simulink model "B733_SAS"  (R2018a)
settings: Solver=VariableStepAuto  StartTime=0.0  StopTime=S.simtime  RelTol=1e-3
undefined symbols (not defined in the file): S
libraries: peGeneralControl x1
settings Model: Creator=Can Bekar  LastModifiedBy=Can Bekar
settings DataIOCC: ExternalInput=S.usignal  InitialState=xu  LoadExternalInput=on  SignalLogging=off  DSMLogging=off

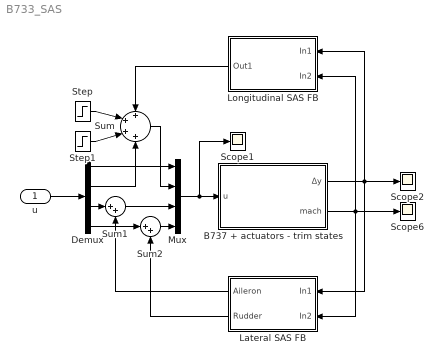
== system B733_SAS ==
  u : Inport
  B737 + actuators - trim states : Subsystem
  Demux : Demux
  Lateral SAS FB : Subsystem
  Longitudinal SAS FB : Subsystem
  Mux : Mux
  Scope1 : Scope
  Scope2 : Scope
  Scope6 : Scope
  Step : Step  Time=2  Before=deg2rad(1)  After=deg2rad(-1)  SampleTime=0
  Step1 : Step  After=deg2rad(1)  SampleTime=0
  Sum : Sum  Inputs=++++
  Sum1 : Sum  Inputs=|++
  Sum2 : Sum  Inputs=|++
  wires:
  Demux/1 -> Mux/1
  Sum/1 -> Mux/2
  Demux/2 -> Sum/4
  Mux/1 -> Scope1/1, B737 + actuators - trim states/1(u)
  u/1 -> Demux/1
  Step1/1 -> Sum/3
  Step/1 -> Sum/2
  Sum1/1 -> Mux/3
  Demux/3 -> Sum1/1
  Sum2/1 -> Mux/4
  Demux/4 -> Sum2/1
  B737 + actuators - trim states/1(Δy) -> Lateral SAS FB/1(In1), Scope2/1, Longitudinal SAS FB/1(In1)
  B737 + actuators - trim states/2(mach) -> Lateral SAS FB/2(In2), Longitudinal SAS FB/2(In2), Scope6/1
  Longitudinal SAS FB/1(Out1) -> Sum/1
  Lateral SAS FB/1(Aileron) -> Sum1/2
  Lateral SAS FB/2(Rudder) -> Sum2/2

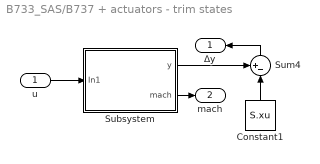
== system B733_SAS/B737 + actuators - trim states ==
  u : Inport
  Constant1 : Constant  Value=S.xu
  Subsystem : Subsystem
  Sum4 : Sum  Inputs=+-|
  Δy : Outport
  mach : Outport  Port=2
  wires:
  Sum4/1 -> Δy/1
  Subsystem/1(y) -> Sum4/1
  u/1 -> Subsystem/1(In1)
  Constant1/1 -> Sum4/2
  Subsystem/2(mach) -> mach/1

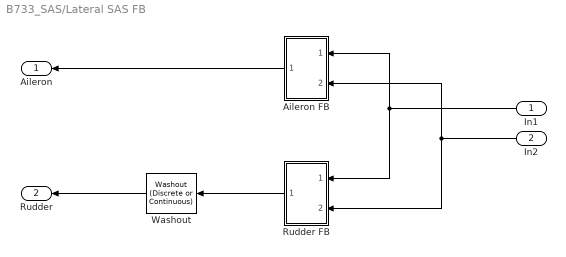
== system B733_SAS/Lateral SAS FB ==
  In1 : Inport
  In2 : Inport  Port=2
  Aileron FB : Subsystem
  Rudder FB : Subsystem
  Washout : peGeneralControl/Washout (Discrete or Continuous)  T=1  Ts=-1
  Aileron : Outport
  Rudder : Outport  Port=2
  wires:
  Washout/1 -> Rudder/1
  In2/1 -> Rudder FB/2(In2), Aileron FB/2(In2)
  In1/1 -> Rudder FB/1(In1), Aileron FB/1(In1)
  Aileron FB/1(Out1) -> Aileron/1
  Rudder FB/1(Out1) -> Washout/1

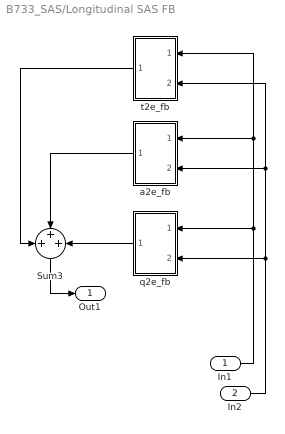
== system B733_SAS/Longitudinal SAS FB ==
  In1 : Inport
  In2 : Inport  Port=2
  Sum3 : Sum  Inputs=+++
  a2e_fb : Subsystem
  q2e_fb : Subsystem
  t2e_fb : Subsystem
  Out1 : Outport
  wires:
  t2e_fb/1(Out1) -> Sum3/1
  Sum3/1 -> Out1/1
  In2/1 -> a2e_fb/2(In2), t2e_fb/2(In2), q2e_fb/2(In2)
  In1/1 -> q2e_fb/1(In1), a2e_fb/1(In1), t2e_fb/1(In1)
  a2e_fb/1(Out1) -> Sum3/2
  q2e_fb/1(Out1) -> Sum3/3

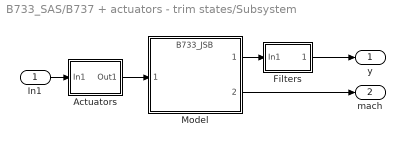
== system B733_SAS/B737 + actuators - trim states/Subsystem ==
  In1 : Inport
  Actuators : Subsystem
  Filters : Subsystem
  Model : ModelReference  ModelNameDialog=B733_JSB  SimulationMode=Normal  ModelReferenceVersion=1.186
  y : Outport
  mach : Outport  Port=2
  wires:
  Model/2 -> mach/1
  Model/1 -> Filters/1(In1)
  Filters/1(Out1) -> y/1
  In1/1 -> Actuators/1(In1)
  Actuators/1(Out1) -> Model/1

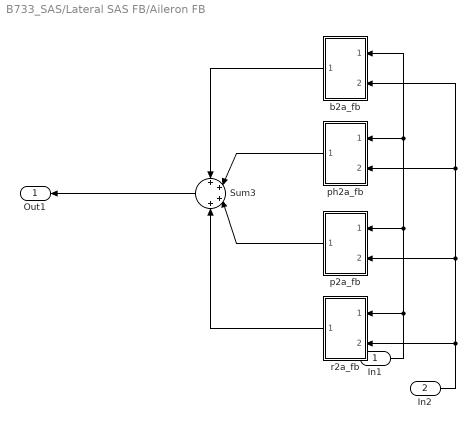
== system B733_SAS/Lateral SAS FB/Aileron FB ==
  In1 : Inport
  In2 : Inport  Port=2
  Sum3 : Sum  Inputs=++++
  b2a_fb : Subsystem
  p2a_fb : Subsystem
  ph2a_fb : Subsystem
  r2a_fb : Subsystem
  Out1 : Outport
  wires:
  p2a_fb/1(Out1) -> Sum3/3
  ph2a_fb/1(Out1) -> Sum3/2
  In2/1 -> b2a_fb/2(In2), ph2a_fb/2(In2), p2a_fb/2(In2), r2a_fb/2(In2)
  b2a_fb/1(Out1) -> Sum3/1
  In1/1 -> b2a_fb/1(In1), ph2a_fb/1(In1), p2a_fb/1(In1), r2a_fb/1(In1)
  r2a_fb/1(Out1) -> Sum3/4
  Sum3/1 -> Out1/1

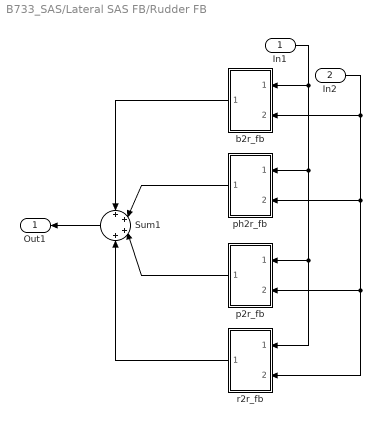
== system B733_SAS/Lateral SAS FB/Rudder FB ==
  In1 : Inport
  In2 : Inport  Port=2
  Sum1 : Sum  Inputs=++++
  b2r_fb : Subsystem
  p2r_fb : Subsystem
  ph2r_fb : Subsystem
  r2r_fb : Subsystem
  Out1 : Outport
  wires:
  r2r_fb/1(Out1) -> Sum1/4
  In2/1 -> ph2r_fb/2(In2), p2r_fb/2(In2), r2r_fb/2(In2), b2r_fb/2(In2)
  b2r_fb/1(Out1) -> Sum1/1
  In1/1 -> ph2r_fb/1(In1), p2r_fb/1(In1), r2r_fb/1(In1), b2r_fb/1(In1)
  p2r_fb/1(Out1) -> Sum1/3
  ph2r_fb/1(Out1) -> Sum1/2
  Sum1/1 -> Out1/1

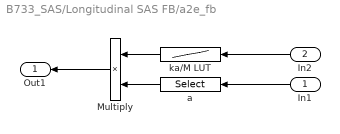
== system B733_SAS/Longitudinal SAS FB/a2e_fb ==
  In1 : Inport
  In2 : Inport  Port=2
  Multiply : Product
  a : Selector  InputPortWidth=12  IndexOptions=Index vector (dialog)  Indices=[2]  OutputSizes=1
  ka/M LUT : Lookup_n-D  NumberOfTableDimensions=1  BreakpointsForDimension1=S.M'  Table=S.kaLUT  InternalRulePriority=Speed  RndMeth=Simplest  InputSameDT=on
  Out1 : Outport
  wires:
  Multiply/1 -> Out1/1
  ka/M LUT/1 -> Multiply/1
  In2/1 -> ka/M LUT/1
  In1/1 -> a/1
  a/1 -> Multiply/2

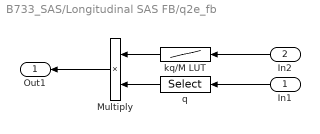
== system B733_SAS/Longitudinal SAS FB/q2e_fb ==
  In1 : Inport
  In2 : Inport  Port=2
  Multiply : Product
  kq/M LUT : Lookup_n-D  NumberOfTableDimensions=1  BreakpointsForDimension1=S.M'  Table=S.kqLUT  InternalRulePriority=Speed  RndMeth=Simplest  InputSameDT=on
  q : Selector  InputPortWidth=12  IndexOptions=Index vector (dialog)  Indices=[8]  OutputSizes=1
  Out1 : Outport
  wires:
  q/1 -> Multiply/2
  In1/1 -> q/1
  In2/1 -> kq/M LUT/1
  kq/M LUT/1 -> Multiply/1
  Multiply/1 -> Out1/1

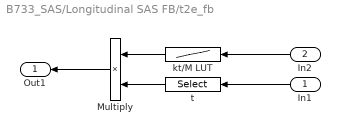
== system B733_SAS/Longitudinal SAS FB/t2e_fb ==
  In1 : Inport
  In2 : Inport  Port=2
  Multiply : Product
  kt/M LUT : Lookup_n-D  NumberOfTableDimensions=1  BreakpointsForDimension1=S.M'  Table=S.ktLUT  InternalRulePriority=Speed  RndMeth=Simplest  InputSameDT=on
  t : Selector  InputPortWidth=12  IndexOptions=Index vector (dialog)  Indices=[5]  OutputSizes=1
  Out1 : Outport
  wires:
  t/1 -> Multiply/2
  In1/1 -> t/1
  In2/1 -> kt/M LUT/1
  kt/M LUT/1 -> Multiply/1
  Multiply/1 -> Out1/1

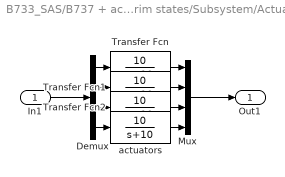
== system B733_SAS/B737 + actuators - trim states/Subsystem/Actuators ==
  In1 : Inport
  Demux : Demux
  Mux : Mux
  Transfer Fcn : TransferFcn  Numerator=[10]  Denominator=[1 10]
  Transfer Fcn1 : TransferFcn  Numerator=[10]  Denominator=[1 10]
  Transfer Fcn2 : TransferFcn  Numerator=[10]  Denominator=[1 10]
  actuators : TransferFcn  Numerator=[10]  Denominator=[1 10]
  Out1 : Outport
  wires:
  actuators/1 -> Mux/4
  Transfer Fcn/1 -> Mux/1
  In1/1 -> Demux/1
  Demux/2 -> Transfer Fcn1/1
  Transfer Fcn1/1 -> Mux/2
  Demux/3 -> Transfer Fcn2/1
  Transfer Fcn2/1 -> Mux/3
  Demux/4 -> actuators/1
  Demux/1 -> Transfer Fcn/1
  Mux/1 -> Out1/1

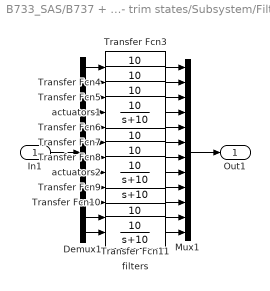
== system B733_SAS/B737 + actuators - trim states/Subsystem/Filters ==
  In1 : Inport
  Demux1 : Demux  Outputs=12
  Mux1 : Mux  Inputs=12
  Transfer Fcn{3..11} (9 alike) : TransferFcn  Numerator=[10]  Denominator=[1 10]
  actuators1 : TransferFcn  Numerator=[10]  Denominator=[1 10]
  actuators2 : TransferFcn  Numerator=[10]  Denominator=[1 10]
  filters : TransferFcn  Numerator=[10]  Denominator=[1 10]
  Out1 : Outport
  wires:
  Demux1/11 -> Transfer Fcn11/1
  Transfer Fcn8/1 -> Mux1/7
  Transfer Fcn4/1 -> Mux1/2
  filters/1 -> Mux1/12
  Demux1/3 -> Transfer Fcn5/1
  Transfer Fcn7/1 -> Mux1/6
  Demux1/12 -> filters/1
  actuators1/1 -> Mux1/4
  Transfer Fcn3/1 -> Mux1/1
  Transfer Fcn11/1 -> Mux1/11
  In1/1 -> Demux1/1
  Demux1/9 -> Transfer Fcn9/1
  Transfer Fcn6/1 -> Mux1/5
  Demux1/1 -> Transfer Fcn3/1
  Demux1/4 -> actuators1/1
  Transfer Fcn5/1 -> Mux1/3
  Demux1/2 -> Transfer Fcn4/1
  Demux1/8 -> actuators2/1
  Transfer Fcn10/1 -> Mux1/10
  Demux1/10 -> Transfer Fcn10/1
  Transfer Fcn9/1 -> Mux1/9
  Demux1/5 -> Transfer Fcn6/1
  Demux1/6 -> Transfer Fcn7/1
  Demux1/7 -> Transfer Fcn8/1
  Mux1/1 -> Out1/1
  actuators2/1 -> Mux1/8

== system B733_SAS/Lateral SAS FB/Aileron FB/b2a_fb ==
  In1 : Inport
  In2 : Inport  Port=2
  Multiply : Product
  kb/M LUT : Lookup_n-D  NumberOfTableDimensions=1  BreakpointsForDimension1=S.M'  Table=S.kbLUT  InternalRulePriority=Speed  RndMeth=Simplest  InputSameDT=on
  t : Selector  InputPortWidth=12  IndexOptions=Index vector (dialog)  Indices=[3]  OutputSizes=1
  Out1 : Outport
  wires:
  Multiply/1 -> Out1/1
  kb/M LUT/1 -> Multiply/1
  In2/1 -> kb/M LUT/1
  In1/1 -> t/1
  t/1 -> Multiply/2

== system B733_SAS/Lateral SAS FB/Aileron FB/p2a_fb ==
  In1 : Inport
  In2 : Inport  Port=2
  Multiply : Product
  kp/M LUT : Lookup_n-D  NumberOfTableDimensions=1  BreakpointsForDimension1=S.M'  Table=S.kpLUT  InternalRulePriority=Speed  RndMeth=Simplest  InputSameDT=on
  p : Selector  InputPortWidth=12  IndexOptions=Index vector (dialog)  Indices=[7]  OutputSizes=1
  Out1 : Outport
  wires:
  Multiply/1 -> Out1/1
  kp/M LUT/1 -> Multiply/1
  In2/1 -> kp/M LUT/1
  In1/1 -> p/1
  p/1 -> Multiply/2

== system B733_SAS/Lateral SAS FB/Aileron FB/ph2a_fb ==
  In1 : Inport
  In2 : Inport  Port=2
  Multiply : Product
  kphi/M LUT : Lookup_n-D  NumberOfTableDimensions=1  BreakpointsForDimension1=S.M'  Table=S.kphLUT  InternalRulePriority=Speed  RndMeth=Simplest  InputSameDT=on
  phi : Selector  InputPortWidth=12  IndexOptions=Index vector (dialog)  Indices=[4]  OutputSizes=1
  Out1 : Outport
  wires:
  phi/1 -> Multiply/2
  In1/1 -> phi/1
  In2/1 -> kphi/M LUT/1
  kphi/M LUT/1 -> Multiply/1
  Multiply/1 -> Out1/1

== system B733_SAS/Lateral SAS FB/Aileron FB/r2a_fb ==
  In1 : Inport
  In2 : Inport  Port=2
  Multiply : Product
  kr/M LUT : Lookup_n-D  NumberOfTableDimensions=1  BreakpointsForDimension1=S.M'  Table=S.krLUT  InternalRulePriority=Speed  RndMeth=Simplest  InputSameDT=on
  r : Selector  InputPortWidth=12  IndexOptions=Index vector (dialog)  Indices=[9]  OutputSizes=1
  Out1 : Outport
  wires:
  r/1 -> Multiply/2
  In1/1 -> r/1
  In2/1 -> kr/M LUT/1
  kr/M LUT/1 -> Multiply/1
  Multiply/1 -> Out1/1

== system B733_SAS/Lateral SAS FB/Rudder FB/b2r_fb ==
  In1 : Inport
  In2 : Inport  Port=2
  Multiply : Product
  b : Selector  InputPortWidth=12  IndexOptions=Index vector (dialog)  Indices=[3]  OutputSizes=1
  kb/M LUT : Lookup_n-D  NumberOfTableDimensions=1  BreakpointsForDimension1=S.M'  Table=S.kbLUT2  InternalRulePriority=Speed  RndMeth=Simplest  InputSameDT=on
  Out1 : Outport
  wires:
  b/1 -> Multiply/2
  In1/1 -> b/1
  In2/1 -> kb/M LUT/1
  kb/M LUT/1 -> Multiply/1
  Multiply/1 -> Out1/1

== system B733_SAS/Lateral SAS FB/Rudder FB/p2r_fb ==
  In1 : Inport
  In2 : Inport  Port=2
  Multiply : Product
  kp/M LUT : Lookup_n-D  NumberOfTableDimensions=1  BreakpointsForDimension1=S.M'  Table=S.kpLUT2  InternalRulePriority=Speed  RndMeth=Simplest  InputSameDT=on
  p : Selector  InputPortWidth=12  IndexOptions=Index vector (dialog)  Indices=[7]  OutputSizes=1
  Out1 : Outport
  wires:
  p/1 -> Multiply/2
  In1/1 -> p/1
  In2/1 -> kp/M LUT/1
  kp/M LUT/1 -> Multiply/1
  Multiply/1 -> Out1/1

== system B733_SAS/Lateral SAS FB/Rudder FB/ph2r_fb ==
  In1 : Inport
  In2 : Inport  Port=2
  Multiply : Product
  kphi/M LUT : Lookup_n-D  NumberOfTableDimensions=1  BreakpointsForDimension1=S.M'  Table=S.kphLUT2  InternalRulePriority=Speed  RndMeth=Simplest  InputSameDT=on
  phi : Selector  InputPortWidth=12  IndexOptions=Index vector (dialog)  Indices=[4]  OutputSizes=1
  Out1 : Outport
  wires:
  Multiply/1 -> Out1/1
  kphi/M LUT/1 -> Multiply/1
  In2/1 -> kphi/M LUT/1
  In1/1 -> phi/1
  phi/1 -> Multiply/2

== system B733_SAS/Lateral SAS FB/Rudder FB/r2r_fb ==
  In1 : Inport
  In2 : Inport  Port=2
  Multiply : Product
  kr/M LUT : Lookup_n-D  NumberOfTableDimensions=1  BreakpointsForDimension1=S.M'  Table=S.krLUT2  InternalRulePriority=Speed  RndMeth=Simplest  InputSameDT=on
  r : Selector  InputPortWidth=12  IndexOptions=Index vector (dialog)  Indices=[9]  OutputSizes=1
  Out1 : Outport
  wires:
  Multiply/1 -> Out1/1
  kr/M LUT/1 -> Multiply/1
  In2/1 -> kr/M LUT/1
  In1/1 -> r/1
  r/1 -> Multiply/2
